simulink model "comapracao_baldursson_david"  (R2012b)
settings: Solver=ode8  StartTime=0.0  StopTime=1  FixedStep=1e-5  RelTol=1e-3
undefined symbols (not defined in the file): fcem_a, fcem_b, fcem_c
libraries: simulink x12, BLDC x2
settings Model: Creator=h3now  LastModifiedBy=h3now

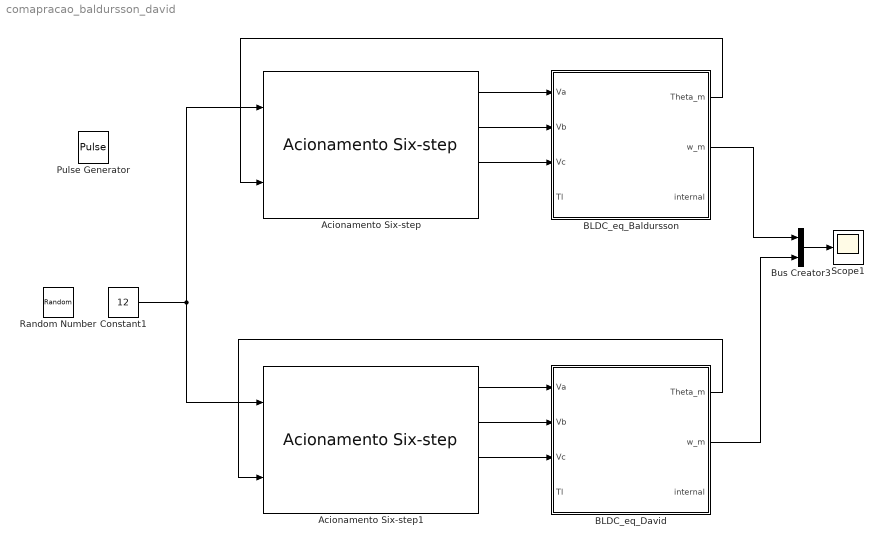
== system comapracao_baldursson_david ==
  Acionamento Six-step : BLDC/Acionamento Six-step  P=8
  Acionamento Six-step1 : BLDC/Acionamento Six-step  P=8
  BLDC_eq_Baldursson : Subsystem  mask(Simulador de um motor BLDC){J=1.39e-6, R=10.1/2, L=2.04/2000, P=8, Kt=15.7e-3/1.19, Ke=15.7e-3/1.19, Kd=0, default_fcem=on, fcem_a=fcem_a, fcem_b=fcem_b, fcem_c=fcem_c}
      mask prompts: J "Inércia do sistema motor+carga [Kg.m^2]"; R "Resistência por fase [Ohm]"; L "Indutância por fase [Henry]"; P "Número de pólos"; Kt "Constante de torque [Nm/A]"; Ke "Constante de força eletromotriz [V.s] (numericamente igual à constante de torque se utilizar SI)"; Kd "Constante de atrito viscoso"; default_fcem "Utilizar back-emf trapezoidal?"; fcem_a "Lookup table da back-emf fase a"; fcem_b "Lookup table da back-emf fase b"; fcem_c "Lookup table da back-emf fase c"
      mask help:
      | Entradas
      | - Vx: tensões na fase 'x' [V]
      | - Tl: torque da carga [N.m]
      |
      | Saídas
      | - Theta_m: ângulo do rotor [rad]
      | - w_m: velocidade ângular do rotor [rad/s]
      | - internal: vetor de variáveis internas do simulador:
      |     - FCEM em cada fase [V] (3x1)
      |     - Corrente em cada fase [A] (3x1)
      |     - Torque produzido por cada fase [N.m] (3x1)
      |     - Torque total [N.m] (1x1)
      mask init:
      | % Se o usuário escolheu utilizar a back-emf padrão, inicializa as variáveis
      | % da lookuptables com valores zerados para não dar erro.
      | if default_fcem == 1
      |     fcem_a = [0,0;1,0];
      |     fcem_b = [0,0;1,0];
      |     fcem_c = [0,0;1,0];
      |     
      | % Se o usuário escolheu especificar qual será a forma da back-emf, checa se
      | % as lookup tables que ele inseriu fazem sentido.
      | else
      |     % Checa se a primeira coluna começa em 0.
      |     if fcem_a(1,1) ~= 0 ||fcem_b(1,1) ~= 0 || fcem_c(1,1) ~= 0
      |         error('A primeira coluna das lookup tables que definem o formato da back-emf devem começar em zero!');
      |     end
      |     % Checa se a primeira coluna termina em 360.
      |     if fcem_a(size(fcem_a,1),1) ~= 360 || fcem_b(size(fcem_b,1),1) ~= 360 || fcem_c(size(fcem_c,1),1) ~= 360
      |         error('A primeira coluna das lookup tables que definem o formato da back-emf deve terminar em 360!');
      |     end
      | end
      mask Callback default_fcem:
      | maskStr = get_param(gcb,'MaskValues');
      | 
      | if strcmp(maskStr{8},'on')
      |     set_param(gcb,'MaskVisibilities',{'on';'on';'on';'on';'on';'on';'on';'on';'off';'off';'off'});
      | else
      |     set_param(gcb,'MaskVisibilities',{'on';'on';'on';'on';'on';'on';'on';'on';'on';'on';'on'});
      | end
  BLDC_eq_David : Subsystem  mask(Simulador de um motor BLDC){J=1.39e-6, R=10.1/2, L=2.04/2000, P=8, Kt=15.7e-3/1.19, Ke=15.7e-3/1.19, Kd=0, default_fcem=on, fcem_a=fcem_a, fcem_b=fcem_b, fcem_c=fcem_c}
      mask prompts: J "Inércia do sistema motor+carga [Kg.m^2]"; R "Resistência por fase [Ohm]"; L "Indutância por fase [Henry]"; P "Número de pólos"; Kt "Constante de torque [Nm/A]"; Ke "Constante de força eletromotriz [V.s] (numericamente igual à constante de torque se utilizar SI)"; Kd "Constante de atrito viscoso"; default_fcem "Utilizar back-emf trapezoidal?"; fcem_a "Lookup table da back-emf fase a"; fcem_b "Lookup table da back-emf fase b"; fcem_c "Lookup table da back-emf fase c"
      mask help:
      | Entradas
      | - Vx: tensões na fase 'x' [V]
      | - Tl: torque da carga [N.m]
      |
      | Saídas
      | - Theta_m: ângulo do rotor [rad]
      | - w_m: velocidade ângular do rotor [rad/s]
      | - internal: vetor de variáveis internas do simulador:
      |     - FCEM em cada fase [V] (3x1)
      |     - Corrente em cada fase [A] (3x1)
      |     - Torque produzido por cada fase [N.m] (3x1)
      |     - Torque total [N.m] (1x1)
      mask init: same as comapracao_baldursson_david/BLDC_eq_Baldursson
      mask Callback default_fcem:
      | maskStr = get_param(gcb,'MaskValues');
      | 
      | if strcmp(maskStr{8},'on')
      |     set_param(gcb,'MaskVisibilities',{'on';'on';'on';'on';'on';'on';'on';'on';'off';'off';'off'});
      | else
      |     set_param(gcb,'MaskVisibilities',{'on';'on';'on';'on';'on';'on';'on';'on';'on';'on';'on'});
      | end
  Bus Creator3 : BusCreator  Inputs=2
  Constant1 : Constant  Value=12
  Pulse Generator : DiscretePulseGenerator  PulseType=Time based  Amplitude=12  Period=1  PulseWidth=50
  Random Number : RandomNumber  Mean=12  Variance=100  SampleTime=0.5
  Scope1 : Scope
      settings: TimeRange=0.35  YMin=-2e+303  YMax=1.2e+304
  wires:
  Acionamento Six-step/1 -> BLDC_eq_Baldursson/1(Va)
  Acionamento Six-step/2 -> BLDC_eq_Baldursson/2(Vb)
  Acionamento Six-step/3 -> BLDC_eq_Baldursson/3(Vc)
  BLDC_eq_Baldursson/1(Theta_m) -> Acionamento Six-step/2
  BLDC_eq_David/1(Theta_m) -> Acionamento Six-step1/2
  Constant1/1 -> Acionamento Six-step/1, Acionamento Six-step1/1
  Bus Creator3/1 -> Scope1/1
  BLDC_eq_Baldursson/2(w_m) -> Bus Creator3/1
  BLDC_eq_David/2(w_m) -> Bus Creator3/2
  Acionamento Six-step1/1 -> BLDC_eq_David/1(Va)
  Acionamento Six-step1/2 -> BLDC_eq_David/2(Vb)
  Acionamento Six-step1/3 -> BLDC_eq_David/3(Vc)

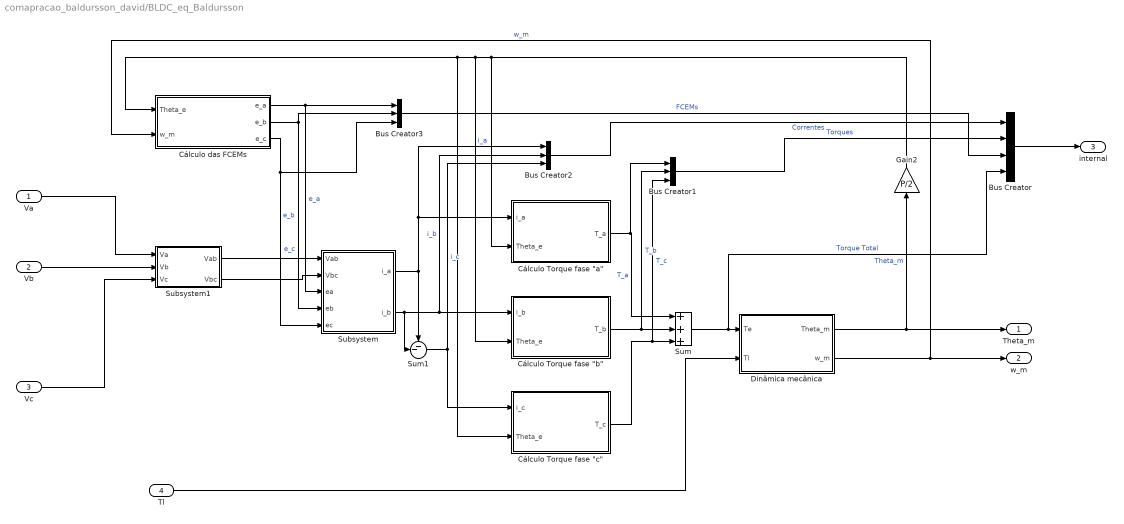
== system comapracao_baldursson_david/BLDC_eq_Baldursson ==
  Va : Inport
  Vb : Inport  Port=2
  Vc : Inport  Port=3
  Tl : Inport  Port=4
  Bus Creator : BusCreator
  Bus Creator1 : BusCreator  Inputs=3
  Bus Creator2 : BusCreator  Inputs=3
  Bus Creator3 : BusCreator  Inputs=3
  "Cálculo Torque fase \"a\"" : Subsystem
  "Cálculo Torque fase \"b\"" : Subsystem
  "Cálculo Torque fase \"c\"" : Subsystem
  Cálculo das FCEMs : Subsystem
  "Dinâmica mecânica " : Subsystem
  Gain2 : Gain  Gain=P/2
  Subsystem : Subsystem
  Subsystem1 : Subsystem
  Sum : Sum  Inputs=+++
  Sum1 : Sum  Inputs=--|
  Theta_m : Outport
  w_m : Outport  Port=2
  internal : Outport  Port=3
  wires:
  Bus Creator1/1 -> Bus Creator/2  "Torques"
  Bus Creator2/1 -> Bus Creator/1  "Correntes"
  Bus Creator3/1 -> Bus Creator/3  "FCEMs"
  Bus Creator/1 -> internal/1
  Cálculo das FCEMs/1(e_a) -> Bus Creator3/1, Subsystem/3(ea)  "e_a"
  Cálculo das FCEMs/2(e_b) -> Subsystem/4(eb), Bus Creator3/2  "e_b"
  Cálculo das FCEMs/3(e_c) -> Subsystem/5(ec), Bus Creator3/3  "e_c"
  Va/1 -> Subsystem1/1(Va)
  Vb/1 -> Subsystem1/2(Vb)
  Vc/1 -> Subsystem1/3(Vc)
  Subsystem/1(i_a) -> Sum1/1, "Cálculo Torque fase \"a\""/1(i_a), Bus Creator2/1  "i_a"
  Subsystem/2(i_b) -> Sum1/2, "Cálculo Torque fase \"b\""/1(i_b), Bus Creator2/2  "i_b"
  Sum1/1 -> "Cálculo Torque fase \"c\""/1(i_c), Bus Creator2/3  "i_c"
  "Cálculo Torque fase \"a\""/1(T_a) -> Sum/1, Bus Creator1/1  "T_a"
  "Cálculo Torque fase \"b\""/1(T_b) -> Sum/2, Bus Creator1/2  "T_b"
  "Cálculo Torque fase \"c\""/1(T_c) -> Sum/3, Bus Creator1/3  "T_c"
  Sum/1 -> "Dinâmica mecânica "/1(Te), Bus Creator/4  "Torque Total"
  "Dinâmica mecânica "/1(Theta_m) -> Theta_m/1, Gain2/1  "Theta_m"
  "Dinâmica mecânica "/2(w_m) -> Cálculo das FCEMs/2(w_m), w_m/1  "w_m"
  Tl/1 -> "Dinâmica mecânica "/2(Tl)
  Gain2/1 -> "Cálculo Torque fase \"a\""/2(Theta_e), "Cálculo Torque fase \"c\""/2(Theta_e), Cálculo das FCEMs/1(Theta_e), "Cálculo Torque fase \"b\""/2(Theta_e)
  Subsystem1/1(Vab) -> Subsystem/1(Vab)
  Subsystem1/2(Vbc) -> Subsystem/2(Vbc)

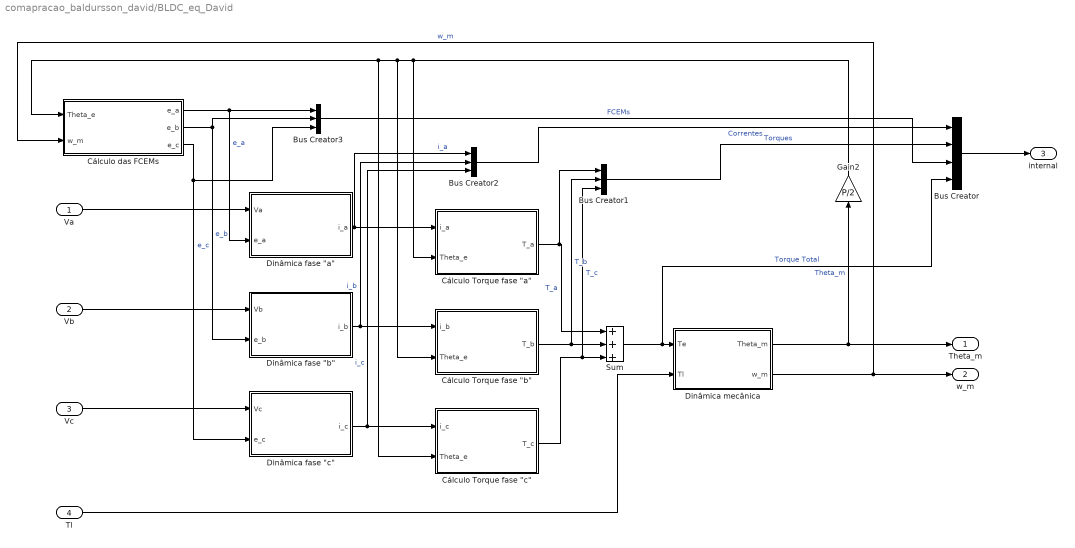
== system comapracao_baldursson_david/BLDC_eq_David ==
  Va : Inport
  Vb : Inport  Port=2
  Vc : Inport  Port=3
  Tl : Inport  Port=4
  Bus Creator : BusCreator
  Bus Creator1 : BusCreator  Inputs=3
  Bus Creator2 : BusCreator  Inputs=3
  Bus Creator3 : BusCreator  Inputs=3
  "Cálculo Torque fase \"a\"" : Subsystem
  "Cálculo Torque fase \"b\"" : Subsystem
  "Cálculo Torque fase \"c\"" : Subsystem
  Cálculo das FCEMs : Subsystem
  "Dinâmica fase \"a\"" : Subsystem
  "Dinâmica fase \"b\"" : Subsystem
  "Dinâmica fase \"c\"" : Subsystem
  "Dinâmica mecânica " : Subsystem
  Gain2 : Gain  Gain=P/2
  Sum : Sum  Inputs=+++
  Theta_m : Outport
  w_m : Outport  Port=2
  internal : Outport  Port=3
  wires:
  Gain2/1 -> "Cálculo Torque fase \"b\""/2(Theta_e), Cálculo das FCEMs/1(Theta_e), "Cálculo Torque fase \"c\""/2(Theta_e), "Cálculo Torque fase \"a\""/2(Theta_e)
  Tl/1 -> "Dinâmica mecânica "/2(Tl)
  "Dinâmica mecânica "/2(w_m) -> w_m/1, Cálculo das FCEMs/2(w_m)  "w_m"
  "Dinâmica mecânica "/1(Theta_m) -> Gain2/1, Theta_m/1  "Theta_m"
  Sum/1 -> Bus Creator/4, "Dinâmica mecânica "/1(Te)  "Torque Total"
  "Cálculo Torque fase \"c\""/1(T_c) -> Bus Creator1/3, Sum/3  "T_c"
  "Cálculo Torque fase \"b\""/1(T_b) -> Bus Creator1/2, Sum/2  "T_b"
  "Cálculo Torque fase \"a\""/1(T_a) -> Bus Creator1/1, Sum/1  "T_a"
  "Dinâmica fase \"c\""/1(i_c) -> Bus Creator2/3, "Cálculo Torque fase \"c\""/1(i_c)  "i_c"
  "Dinâmica fase \"b\""/1(i_b) -> Bus Creator2/2, "Cálculo Torque fase \"b\""/1(i_b)  "i_b"
  "Dinâmica fase \"a\""/1(i_a) -> Bus Creator2/1, "Cálculo Torque fase \"a\""/1(i_a)  "i_a"
  Vc/1 -> "Dinâmica fase \"c\""/1(Vc)
  Vb/1 -> "Dinâmica fase \"b\""/1(Vb)
  Va/1 -> "Dinâmica fase \"a\""/1(Va)
  Cálculo das FCEMs/3(e_c) -> Bus Creator3/3, "Dinâmica fase \"c\""/2(e_c)  "e_c"
  Cálculo das FCEMs/2(e_b) -> "Dinâmica fase \"b\""/2(e_b), Bus Creator3/2  "e_b"
  Cálculo das FCEMs/1(e_a) -> "Dinâmica fase \"a\""/2(e_a), Bus Creator3/1  "e_a"
  Bus Creator/1 -> internal/1
  Bus Creator3/1 -> Bus Creator/3  "FCEMs"
  Bus Creator2/1 -> Bus Creator/1  "Correntes"
  Bus Creator1/1 -> Bus Creator/2  "Torques"

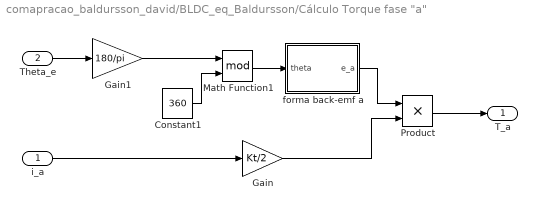
== system comapracao_baldursson_david/BLDC_eq_Baldursson/Cálculo Torque fase "a" ==
  i_a : Inport
  Theta_e : Inport  Port=2
  Constant1 : Constant  Value=360
  Gain : Gain  Gain=Kt/2
  Gain1 : Gain  Gain=180/pi
  Math Function1 : Math  Operator=mod  SaturateOnIntegerOverflow=on
  Product : Product  RndMeth=Zero
  forma back-emf a : Subsystem
  T_a : Outport
  wires:
  i_a/1 -> Gain/1
  Gain/1 -> Product/2
  Math Function1/1 -> forma back-emf a/1(theta)
  Theta_e/1 -> Gain1/1
  forma back-emf a/1(e_a) -> Product/1
  Product/1 -> T_a/1
  Gain1/1 -> Math Function1/1
  Constant1/1 -> Math Function1/2

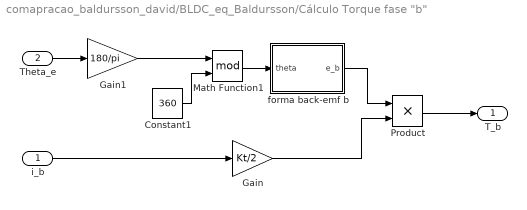
== system comapracao_baldursson_david/BLDC_eq_Baldursson/Cálculo Torque fase "b" ==
  i_b : Inport
  Theta_e : Inport  Port=2
  Constant1 : Constant  Value=360
  Gain : Gain  Gain=Kt/2
  Gain1 : Gain  Gain=180/pi
  Math Function1 : Math  Operator=mod  SaturateOnIntegerOverflow=on
  Product : Product  RndMeth=Zero
  forma back-emf b : Subsystem
  T_b : Outport
  wires:
  Product/1 -> T_b/1
  forma back-emf b/1(e_b) -> Product/1
  Theta_e/1 -> Gain1/1
  Math Function1/1 -> forma back-emf b/1(theta)
  Gain/1 -> Product/2
  i_b/1 -> Gain/1
  Gain1/1 -> Math Function1/1
  Constant1/1 -> Math Function1/2

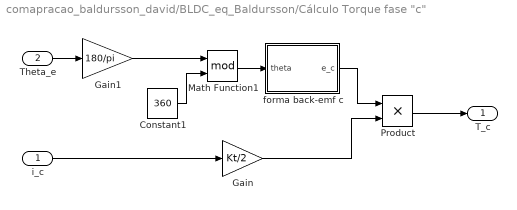
== system comapracao_baldursson_david/BLDC_eq_Baldursson/Cálculo Torque fase "c" ==
  i_c : Inport
  Theta_e : Inport  Port=2
  Constant1 : Constant  Value=360
  Gain : Gain  Gain=Kt/2
  Gain1 : Gain  Gain=180/pi
  Math Function1 : Math  Operator=mod  SaturateOnIntegerOverflow=on
  Product : Product  RndMeth=Zero
  forma back-emf c : Subsystem
  T_c : Outport
  wires:
  i_c/1 -> Gain/1
  Gain/1 -> Product/2
  Math Function1/1 -> forma back-emf c/1(theta)
  Theta_e/1 -> Gain1/1
  forma back-emf c/1(e_c) -> Product/1
  Product/1 -> T_c/1
  Gain1/1 -> Math Function1/1
  Constant1/1 -> Math Function1/2

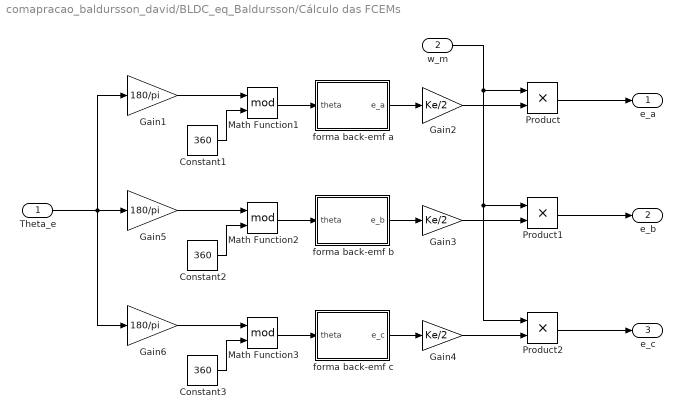
== system comapracao_baldursson_david/BLDC_eq_Baldursson/Cálculo das FCEMs ==
  Theta_e : Inport
  w_m : Inport  Port=2
  Constant1 : Constant  Value=360
  Constant2 : Constant  Value=360
  Constant3 : Constant  Value=360
  Gain1 : Gain  Gain=180/pi
  Gain2 : Gain  Gain=Ke/2
  Gain3 : Gain  Gain=Ke/2
  Gain4 : Gain  Gain=Ke/2
  Gain5 : Gain  Gain=180/pi
  Gain6 : Gain  Gain=180/pi
  Math Function1 : Math  Operator=mod  SaturateOnIntegerOverflow=on
  Math Function2 : Math  Operator=mod  SaturateOnIntegerOverflow=on
  Math Function3 : Math  Operator=mod  SaturateOnIntegerOverflow=on
  Product : Product  RndMeth=Zero
  Product1 : Product  RndMeth=Zero
  Product2 : Product  RndMeth=Zero
  forma back-emf a : Subsystem
  forma back-emf b : Subsystem
  forma back-emf c : Subsystem
  e_a : Outport
  e_b : Outport  Port=2
  e_c : Outport  Port=3
  wires:
  forma back-emf c/1(e_c) -> Gain4/1
  Math Function3/1 -> forma back-emf c/1(theta)
  forma back-emf b/1(e_b) -> Gain3/1
  Math Function2/1 -> forma back-emf b/1(theta)
  forma back-emf a/1(e_a) -> Gain2/1
  Math Function1/1 -> forma back-emf a/1(theta)
  Gain6/1 -> Math Function3/1
  Gain5/1 -> Math Function2/1
  Gain1/1 -> Math Function1/1
  Gain4/1 -> Product2/2
  Gain3/1 -> Product1/2
  w_m/1 -> Product2/1, Product1/1, Product/1
  Gain2/1 -> Product/2
  Product2/1 -> e_c/1
  Theta_e/1 -> Gain6/1, Gain1/1, Gain5/1
  Product1/1 -> e_b/1
  Product/1 -> e_a/1
  Constant1/1 -> Math Function1/2
  Constant2/1 -> Math Function2/2
  Constant3/1 -> Math Function3/2

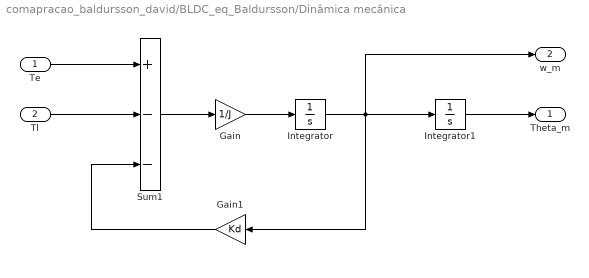
== system comapracao_baldursson_david/BLDC_eq_Baldursson/Dinâmica mecânica  ==
  Te : Inport
  Tl : Inport  Port=2
  Gain : Gain  Gain=1/J
  Gain1 : Gain  Gain=Kd
  Integrator : Integrator
  Integrator1 : Integrator
  Sum1 : Sum  Inputs=+--
  Theta_m : Outport
  w_m : Outport  Port=2
  wires:
  Sum1/1 -> Gain/1
  Gain/1 -> Integrator/1
  Integrator/1 -> w_m/1, Integrator1/1, Gain1/1
  Te/1 -> Sum1/1
  Gain1/1 -> Sum1/3
  Tl/1 -> Sum1/2
  Integrator1/1 -> Theta_m/1

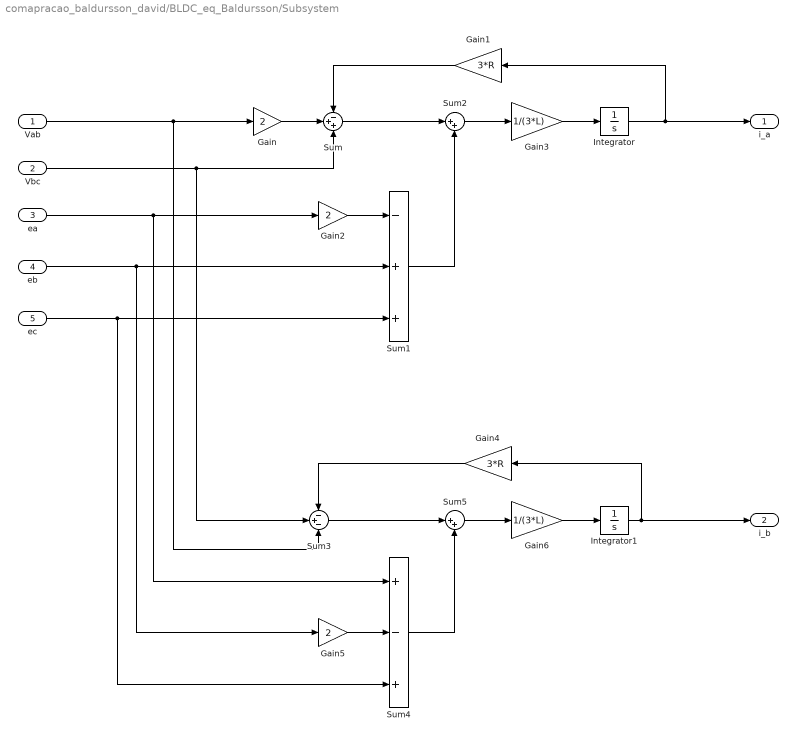
== system comapracao_baldursson_david/BLDC_eq_Baldursson/Subsystem ==
  Vab : Inport
  Vbc : Inport  Port=2
  ea : Inport  Port=3
  eb : Inport  Port=4
  ec : Inport  Port=5
  Gain : Gain  Gain=2
  Gain1 : Gain  Gain=3*R
  Gain2 : Gain  Gain=2
  Gain3 : Gain  Gain=1/(3*L)
  Gain4 : Gain  Gain=3*R
  Gain5 : Gain  Gain=2
  Gain6 : Gain  Gain=1/(3*L)
  Integrator : Integrator
  Integrator1 : Integrator
  Sum : Sum  Inputs=-++
  Sum1 : Sum  Inputs=-++
  Sum2 : Sum  Inputs=|++
  Sum3 : Sum  Inputs=-+-
  Sum4 : Sum  Inputs=+-+
  Sum5 : Sum  Inputs=|++
  i_a : Outport
  i_b : Outport  Port=2
  wires:
  Gain6/1 -> Integrator1/1
  Gain5/1 -> Sum4/2
  Sum3/1 -> Sum5/1
  Sum4/1 -> Sum5/2
  Sum5/1 -> Gain6/1
  Gain2/1 -> Sum1/1
  ea/1 -> Sum4/1, Gain2/1
  Gain1/1 -> Sum/1
  Integrator/1 -> i_a/1, Gain1/1
  Gain/1 -> Sum/2
  Vab/1 -> Sum3/3, Gain/1
  Sum2/1 -> Gain3/1
  Gain3/1 -> Integrator/1
  ec/1 -> Sum4/3, Sum1/3
  eb/1 -> Gain5/1, Sum1/2
  Sum1/1 -> Sum2/2
  Sum/1 -> Sum2/1
  Vbc/1 -> Sum3/2, Sum/3
  Gain4/1 -> Sum3/1
  Integrator1/1 -> i_b/1, Gain4/1

== system comapracao_baldursson_david/BLDC_eq_Baldursson/Subsystem1 ==
  Va : Inport
  Vb : Inport  Port=2
  Vc : Inport  Port=3
  Sum : Sum  Inputs=|+-
  Sum1 : Sum  Inputs=|+-
  Vab : Outport
  Vbc : Outport  Port=2
  wires:
  Va/1 -> Sum/1
  Sum/1 -> Vab/1
  Vb/1 -> Sum1/1, Sum/2
  Vc/1 -> Sum1/2
  Sum1/1 -> Vbc/1

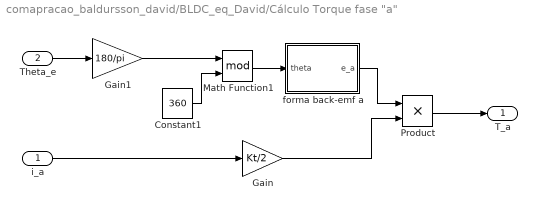
== system comapracao_baldursson_david/BLDC_eq_David/Cálculo Torque fase "a" ==
  i_a : Inport
  Theta_e : Inport  Port=2
  Constant1 : Constant  Value=360
  Gain : Gain  Gain=Kt/2
  Gain1 : Gain  Gain=180/pi
  Math Function1 : Math  Operator=mod  SaturateOnIntegerOverflow=on
  Product : Product  RndMeth=Zero
  forma back-emf a : Subsystem
  T_a : Outport
  wires:
  Constant1/1 -> Math Function1/2
  Gain1/1 -> Math Function1/1
  Product/1 -> T_a/1
  forma back-emf a/1(e_a) -> Product/1
  Theta_e/1 -> Gain1/1
  Math Function1/1 -> forma back-emf a/1(theta)
  Gain/1 -> Product/2
  i_a/1 -> Gain/1

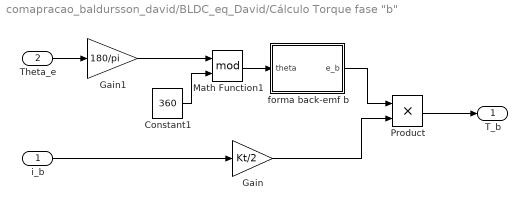
== system comapracao_baldursson_david/BLDC_eq_David/Cálculo Torque fase "b" ==
  i_b : Inport
  Theta_e : Inport  Port=2
  Constant1 : Constant  Value=360
  Gain : Gain  Gain=Kt/2
  Gain1 : Gain  Gain=180/pi
  Math Function1 : Math  Operator=mod  SaturateOnIntegerOverflow=on
  Product : Product  RndMeth=Zero
  forma back-emf b : Subsystem
  T_b : Outport
  wires:
  Constant1/1 -> Math Function1/2
  Gain1/1 -> Math Function1/1
  i_b/1 -> Gain/1
  Gain/1 -> Product/2
  Math Function1/1 -> forma back-emf b/1(theta)
  Theta_e/1 -> Gain1/1
  forma back-emf b/1(e_b) -> Product/1
  Product/1 -> T_b/1

== system comapracao_baldursson_david/BLDC_eq_David/Cálculo Torque fase "c" ==
  i_c : Inport
  Theta_e : Inport  Port=2
  Constant1 : Constant  Value=360
  Gain : Gain  Gain=Kt/2
  Gain1 : Gain  Gain=180/pi
  Math Function1 : Math  Operator=mod  SaturateOnIntegerOverflow=on
  Product : Product  RndMeth=Zero
  forma back-emf c : Subsystem
  T_c : Outport
  wires:
  Constant1/1 -> Math Function1/2
  Gain1/1 -> Math Function1/1
  Product/1 -> T_c/1
  forma back-emf c/1(e_c) -> Product/1
  Theta_e/1 -> Gain1/1
  Math Function1/1 -> forma back-emf c/1(theta)
  Gain/1 -> Product/2
  i_c/1 -> Gain/1

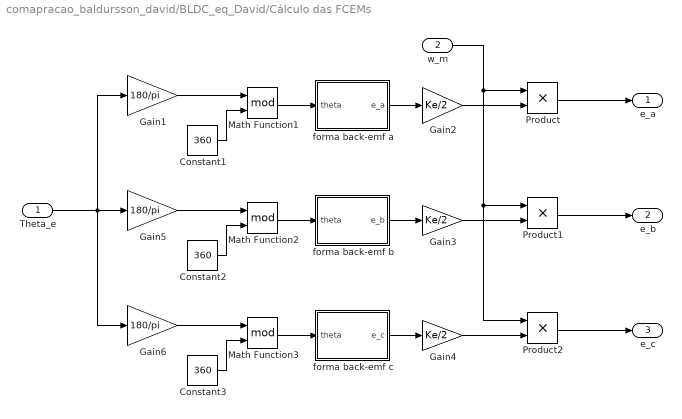
== system comapracao_baldursson_david/BLDC_eq_David/Cálculo das FCEMs ==
  Theta_e : Inport
  w_m : Inport  Port=2
  Constant1 : Constant  Value=360
  Constant2 : Constant  Value=360
  Constant3 : Constant  Value=360
  Gain1 : Gain  Gain=180/pi
  Gain2 : Gain  Gain=Ke/2
  Gain3 : Gain  Gain=Ke/2
  Gain4 : Gain  Gain=Ke/2
  Gain5 : Gain  Gain=180/pi
  Gain6 : Gain  Gain=180/pi
  Math Function1 : Math  Operator=mod  SaturateOnIntegerOverflow=on
  Math Function2 : Math  Operator=mod  SaturateOnIntegerOverflow=on
  Math Function3 : Math  Operator=mod  SaturateOnIntegerOverflow=on
  Product : Product  RndMeth=Zero
  Product1 : Product  RndMeth=Zero
  Product2 : Product  RndMeth=Zero
  forma back-emf a : Subsystem
  forma back-emf b : Subsystem
  forma back-emf c : Subsystem
  e_a : Outport
  e_b : Outport  Port=2
  e_c : Outport  Port=3
  wires:
  Constant3/1 -> Math Function3/2
  Constant2/1 -> Math Function2/2
  Constant1/1 -> Math Function1/2
  Product/1 -> e_a/1
  Product1/1 -> e_b/1
  Theta_e/1 -> Gain5/1, Gain1/1, Gain6/1
  Product2/1 -> e_c/1
  Gain2/1 -> Product/2
  w_m/1 -> Product/1, Product1/1, Product2/1
  Gain3/1 -> Product1/2
  Gain4/1 -> Product2/2
  Gain1/1 -> Math Function1/1
  Gain5/1 -> Math Function2/1
  Gain6/1 -> Math Function3/1
  Math Function1/1 -> forma back-emf a/1(theta)
  forma back-emf a/1(e_a) -> Gain2/1
  Math Function2/1 -> forma back-emf b/1(theta)
  forma back-emf b/1(e_b) -> Gain3/1
  Math Function3/1 -> forma back-emf c/1(theta)
  forma back-emf c/1(e_c) -> Gain4/1

== system comapracao_baldursson_david/BLDC_eq_David/Dinâmica fase "a" ==
  note: Gain
  Va : Inport
  e_a : Inport  Port=2
  " " : Gain  Gain=1/L
  Gain : Gain  Gain=R
  Integrator : Integrator
  Sum : Sum  Inputs=+--
  i_a : Outport
  wires:
  e_a/1 -> Sum/2
  Gain/1 -> Sum/3
  " "/1 -> Integrator/1
  Sum/1 -> " "/1
  Va/1 -> Sum/1
  Integrator/1 -> Gain/1, i_a/1

== system comapracao_baldursson_david/BLDC_eq_David/Dinâmica fase "b" ==
  note: Gain
  Vb : Inport
  e_b : Inport  Port=2
  " " : Gain  Gain=1/L
  Gain : Gain  Gain=R
  Integrator : Integrator
  Sum : Sum  Inputs=+--
  i_b : Outport
  wires:
  Integrator/1 -> i_b/1, Gain/1
  Vb/1 -> Sum/1
  Sum/1 -> " "/1
  " "/1 -> Integrator/1
  Gain/1 -> Sum/3
  e_b/1 -> Sum/2

== system comapracao_baldursson_david/BLDC_eq_David/Dinâmica fase "c" ==
  note: Gain
  Vc : Inport
  e_c : Inport  Port=2
  " " : Gain  Gain=1/L
  Gain : Gain  Gain=R
  Integrator : Integrator
  Sum : Sum  Inputs=+--
  i_c : Outport
  wires:
  e_c/1 -> Sum/2
  Gain/1 -> Sum/3
  " "/1 -> Integrator/1
  Sum/1 -> " "/1
  Vc/1 -> Sum/1
  Integrator/1 -> Gain/1, i_c/1

== system comapracao_baldursson_david/BLDC_eq_David/Dinâmica mecânica  ==
  Te : Inport
  Tl : Inport  Port=2
  Gain : Gain  Gain=1/J
  Gain1 : Gain  Gain=Kd
  Integrator : Integrator
  Integrator1 : Integrator
  Sum1 : Sum  Inputs=+--
  Theta_m : Outport
  w_m : Outport  Port=2
  wires:
  Integrator1/1 -> Theta_m/1
  Tl/1 -> Sum1/2
  Gain1/1 -> Sum1/3
  Te/1 -> Sum1/1
  Integrator/1 -> Gain1/1, Integrator1/1, w_m/1
  Gain/1 -> Integrator/1
  Sum1/1 -> Gain/1

== system comapracao_baldursson_david/BLDC_eq_Baldursson/Cálculo Torque fase "a"/forma back-emf a ==
  theta : Inport
  1-D Lookup Table : Lookup_n-D  NumberOfTableDimensions=1  BreakpointsForDimension1=fcem_a(:,1)  Table=fcem_a(:,2)  RndMeth=Simplest  InputSameDT=on
  Compare To Zero : simulink/Logic and Bit Operations/Compare To Zero  relop=>  OutDataTypeStr=boolean
  Constant : Constant  Value=default_fcem
  Switch : Switch
  fa1 : Lookup  InputValues=[0 30 60 90 120 150 180 210 240 270 300 330 360]  Table=[ 1 1 1 0 -1 -1 -1 -1 -1 0 1 1 1]
  e_a : Outport
  wires:
  Constant/1 -> Compare To Zero/1
  Compare To Zero/1 -> Switch/2
  1-D Lookup Table/1 -> Switch/3
  fa1/1 -> Switch/1
  Switch/1 -> e_a/1
  theta/1 -> fa1/1, 1-D Lookup Table/1

== system comapracao_baldursson_david/BLDC_eq_Baldursson/Cálculo Torque fase "b"/forma back-emf b ==
  theta : Inport
  1-D Lookup Table1 : Lookup_n-D  NumberOfTableDimensions=1  BreakpointsForDimension1=fcem_b(:,1)  Table=fcem_b(:,2)  RndMeth=Simplest  InputSameDT=on
  Compare To Zero1 : simulink/Logic and Bit Operations/Compare To Zero  relop=>  OutDataTypeStr=boolean
  Constant1 : Constant  Value=default_fcem
  Switch : Switch
  fb2 : Lookup  InputValues=[0 30 60 90 120 150 180 210 240 270 300 330 360]  Table=[-1 0 1 1 1 1 1 0 -1 -1 -1 -1 -1]
  e_b : Outport
  wires:
  fb2/1 -> Switch/1
  Switch/1 -> e_b/1
  Constant1/1 -> Compare To Zero1/1
  Compare To Zero1/1 -> Switch/2
  theta/1 -> fb2/1, 1-D Lookup Table1/1
  1-D Lookup Table1/1 -> Switch/3

== system comapracao_baldursson_david/BLDC_eq_Baldursson/Cálculo Torque fase "c"/forma back-emf c ==
  theta : Inport
  1-D Lookup Table : Lookup_n-D  NumberOfTableDimensions=1  BreakpointsForDimension1=fcem_c(:,1)  Table=fcem_c(:,2)  RndMeth=Simplest  InputSameDT=on
  Compare To Zero : simulink/Logic and Bit Operations/Compare To Zero  relop=>  OutDataTypeStr=boolean
  Constant : Constant  Value=default_fcem
  Switch : Switch
  fc1 : Lookup  InputValues=[0 30 60 90 120 150 180 210 240 270 300 330 360]  Table=[-1 -1 -1 -1 -1 0 1 1 1 1 1 0 -1]
  e_c : Outport
  wires:
  fc1/1 -> Switch/1
  Switch/1 -> e_c/1
  Constant/1 -> Compare To Zero/1
  Compare To Zero/1 -> Switch/2
  theta/1 -> fc1/1, 1-D Lookup Table/1
  1-D Lookup Table/1 -> Switch/3

== system comapracao_baldursson_david/BLDC_eq_Baldursson/Cálculo das FCEMs/forma back-emf a ==
  theta : Inport
  1-D Lookup Table : Lookup_n-D  NumberOfTableDimensions=1  BreakpointsForDimension1=fcem_a(:,1)  Table=fcem_a(:,2)  RndMeth=Simplest  InputSameDT=on
  Compare To Zero : simulink/Logic and Bit Operations/Compare To Zero  relop=>  OutDataTypeStr=boolean
  Constant : Constant  Value=default_fcem
  Switch : Switch
  fa1 : Lookup  InputValues=[0 30 60 90 120 150 180 210 240 270 300 330 360]  Table=[ 1 1 1 0 -1 -1 -1 -1 -1 0 1 1 1]
  e_a : Outport
  wires:
  Constant/1 -> Compare To Zero/1
  Compare To Zero/1 -> Switch/2
  1-D Lookup Table/1 -> Switch/3
  fa1/1 -> Switch/1
  Switch/1 -> e_a/1
  theta/1 -> fa1/1, 1-D Lookup Table/1

== system comapracao_baldursson_david/BLDC_eq_Baldursson/Cálculo das FCEMs/forma back-emf b ==
  theta : Inport
  1-D Lookup Table1 : Lookup_n-D  NumberOfTableDimensions=1  BreakpointsForDimension1=fcem_b(:,1)  Table=fcem_b(:,2)  RndMeth=Simplest  InputSameDT=on
  Compare To Zero1 : simulink/Logic and Bit Operations/Compare To Zero  relop=>  OutDataTypeStr=boolean
  Constant1 : Constant  Value=default_fcem
  Switch : Switch
  fb2 : Lookup  InputValues=[0 30 60 90 120 150 180 210 240 270 300 330 360]  Table=[-1 0 1 1 1 1 1 0 -1 -1 -1 -1 -1]
  e_b : Outport
  wires:
  fb2/1 -> Switch/1
  Switch/1 -> e_b/1
  Constant1/1 -> Compare To Zero1/1
  Compare To Zero1/1 -> Switch/2
  theta/1 -> fb2/1, 1-D Lookup Table1/1
  1-D Lookup Table1/1 -> Switch/3

== system comapracao_baldursson_david/BLDC_eq_Baldursson/Cálculo das FCEMs/forma back-emf c ==
  theta : Inport
  1-D Lookup Table : Lookup_n-D  NumberOfTableDimensions=1  BreakpointsForDimension1=fcem_c(:,1)  Table=fcem_c(:,2)  RndMeth=Simplest  InputSameDT=on
  Compare To Zero : simulink/Logic and Bit Operations/Compare To Zero  relop=>  OutDataTypeStr=boolean
  Constant : Constant  Value=default_fcem
  Switch : Switch
  fc1 : Lookup  InputValues=[0 30 60 90 120 150 180 210 240 270 300 330 360]  Table=[-1 -1 -1 -1 -1 0 1 1 1 1 1 0 -1]
  e_c : Outport
  wires:
  fc1/1 -> Switch/1
  Switch/1 -> e_c/1
  Constant/1 -> Compare To Zero/1
  Compare To Zero/1 -> Switch/2
  theta/1 -> fc1/1, 1-D Lookup Table/1
  1-D Lookup Table/1 -> Switch/3

== system comapracao_baldursson_david/BLDC_eq_David/Cálculo Torque fase "a"/forma back-emf a ==
  theta : Inport
  1-D Lookup Table : Lookup_n-D  NumberOfTableDimensions=1  BreakpointsForDimension1=fcem_a(:,1)  Table=fcem_a(:,2)  RndMeth=Simplest  InputSameDT=on
  Compare To Zero : simulink/Logic and Bit Operations/Compare To Zero  relop=>  OutDataTypeStr=boolean
  Constant : Constant  Value=default_fcem
  Switch : Switch
  fa1 : Lookup  InputValues=[0 30 60 90 120 150 180 210 240 270 300 330 360]  Table=[ 1 1 1 0 -1 -1 -1 -1 -1 0 1 1 1]
  e_a : Outport
  wires:
  theta/1 -> 1-D Lookup Table/1, fa1/1
  Switch/1 -> e_a/1
  fa1/1 -> Switch/1
  1-D Lookup Table/1 -> Switch/3
  Compare To Zero/1 -> Switch/2
  Constant/1 -> Compare To Zero/1

== system comapracao_baldursson_david/BLDC_eq_David/Cálculo Torque fase "b"/forma back-emf b ==
  theta : Inport
  1-D Lookup Table1 : Lookup_n-D  NumberOfTableDimensions=1  BreakpointsForDimension1=fcem_b(:,1)  Table=fcem_b(:,2)  RndMeth=Simplest  InputSameDT=on
  Compare To Zero1 : simulink/Logic and Bit Operations/Compare To Zero  relop=>  OutDataTypeStr=boolean
  Constant1 : Constant  Value=default_fcem
  Switch : Switch
  fb2 : Lookup  InputValues=[0 30 60 90 120 150 180 210 240 270 300 330 360]  Table=[-1 0 1 1 1 1 1 0 -1 -1 -1 -1 -1]
  e_b : Outport
  wires:
  1-D Lookup Table1/1 -> Switch/3
  theta/1 -> 1-D Lookup Table1/1, fb2/1
  Compare To Zero1/1 -> Switch/2
  Constant1/1 -> Compare To Zero1/1
  Switch/1 -> e_b/1
  fb2/1 -> Switch/1

== system comapracao_baldursson_david/BLDC_eq_David/Cálculo Torque fase "c"/forma back-emf c ==
  theta : Inport
  1-D Lookup Table : Lookup_n-D  NumberOfTableDimensions=1  BreakpointsForDimension1=fcem_c(:,1)  Table=fcem_c(:,2)  RndMeth=Simplest  InputSameDT=on
  Compare To Zero : simulink/Logic and Bit Operations/Compare To Zero  relop=>  OutDataTypeStr=boolean
  Constant : Constant  Value=default_fcem
  Switch : Switch
  fc1 : Lookup  InputValues=[0 30 60 90 120 150 180 210 240 270 300 330 360]  Table=[-1 -1 -1 -1 -1 0 1 1 1 1 1 0 -1]
  e_c : Outport
  wires:
  1-D Lookup Table/1 -> Switch/3
  theta/1 -> 1-D Lookup Table/1, fc1/1
  Compare To Zero/1 -> Switch/2
  Constant/1 -> Compare To Zero/1
  Switch/1 -> e_c/1
  fc1/1 -> Switch/1

== system comapracao_baldursson_david/BLDC_eq_David/Cálculo das FCEMs/forma back-emf a ==
  theta : Inport
  1-D Lookup Table : Lookup_n-D  NumberOfTableDimensions=1  BreakpointsForDimension1=fcem_a(:,1)  Table=fcem_a(:,2)  RndMeth=Simplest  InputSameDT=on
  Compare To Zero : simulink/Logic and Bit Operations/Compare To Zero  relop=>  OutDataTypeStr=boolean
  Constant : Constant  Value=default_fcem
  Switch : Switch
  fa1 : Lookup  InputValues=[0 30 60 90 120 150 180 210 240 270 300 330 360]  Table=[ 1 1 1 0 -1 -1 -1 -1 -1 0 1 1 1]
  e_a : Outport
  wires:
  theta/1 -> 1-D Lookup Table/1, fa1/1
  Switch/1 -> e_a/1
  fa1/1 -> Switch/1
  1-D Lookup Table/1 -> Switch/3
  Compare To Zero/1 -> Switch/2
  Constant/1 -> Compare To Zero/1

== system comapracao_baldursson_david/BLDC_eq_David/Cálculo das FCEMs/forma back-emf b ==
  theta : Inport
  1-D Lookup Table1 : Lookup_n-D  NumberOfTableDimensions=1  BreakpointsForDimension1=fcem_b(:,1)  Table=fcem_b(:,2)  RndMeth=Simplest  InputSameDT=on
  Compare To Zero1 : simulink/Logic and Bit Operations/Compare To Zero  relop=>  OutDataTypeStr=boolean
  Constant1 : Constant  Value=default_fcem
  Switch : Switch
  fb2 : Lookup  InputValues=[0 30 60 90 120 150 180 210 240 270 300 330 360]  Table=[-1 0 1 1 1 1 1 0 -1 -1 -1 -1 -1]
  e_b : Outport
  wires:
  1-D Lookup Table1/1 -> Switch/3
  theta/1 -> 1-D Lookup Table1/1, fb2/1
  Compare To Zero1/1 -> Switch/2
  Constant1/1 -> Compare To Zero1/1
  Switch/1 -> e_b/1
  fb2/1 -> Switch/1

== system comapracao_baldursson_david/BLDC_eq_David/Cálculo das FCEMs/forma back-emf c ==
  theta : Inport
  1-D Lookup Table : Lookup_n-D  NumberOfTableDimensions=1  BreakpointsForDimension1=fcem_c(:,1)  Table=fcem_c(:,2)  RndMeth=Simplest  InputSameDT=on
  Compare To Zero : simulink/Logic and Bit Operations/Compare To Zero  relop=>  OutDataTypeStr=boolean
  Constant : Constant  Value=default_fcem
  Switch : Switch
  fc1 : Lookup  InputValues=[0 30 60 90 120 150 180 210 240 270 300 330 360]  Table=[-1 -1 -1 -1 -1 0 1 1 1 1 1 0 -1]
  e_c : Outport
  wires:
  1-D Lookup Table/1 -> Switch/3
  theta/1 -> 1-D Lookup Table/1, fc1/1
  Compare To Zero/1 -> Switch/2
  Constant/1 -> Compare To Zero/1
  Switch/1 -> e_c/1
  fc1/1 -> Switch/1
